simulink model "modeling1"  (R2017b)
settings: Solver=FixedStepAuto  StartTime=0.0  StopTime=100.0  FixedStep=0.01  RelTol=1e-3
settings Model: Creator=aokly  LastModifiedBy=aokly

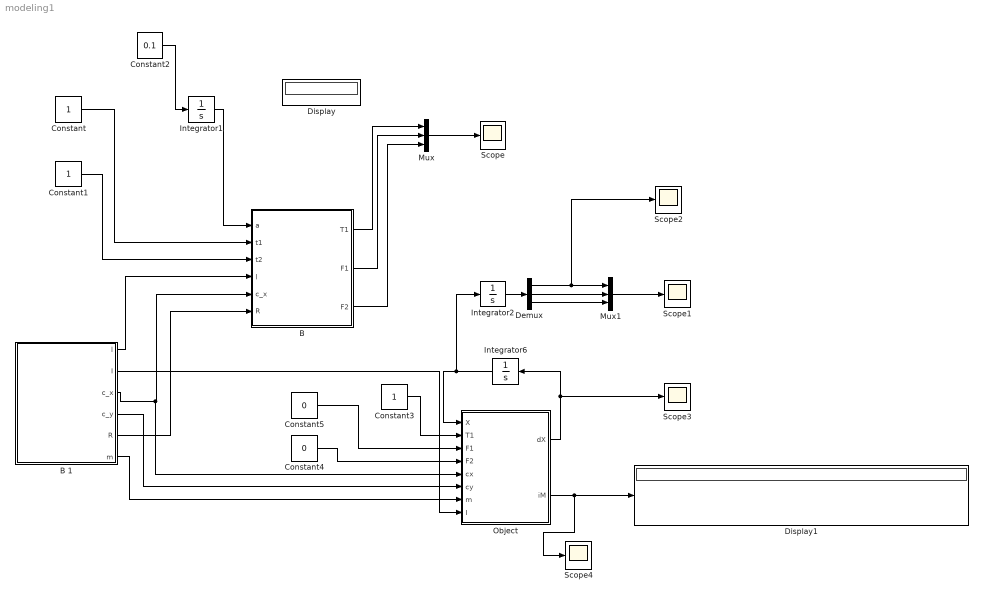
== system modeling1 ==
  "B " : MATLAB Function  TreatAsAtomicUnit=on
  B 1 : MATLAB Function  TreatAsAtomicUnit=on
  Constant : Constant
  Constant1 : Constant
  Constant2 : Constant  Value=0.1
  Constant3 : Constant
  Constant4 : Constant  Value=0
  Constant5 : Constant  Value=0
  Demux : Demux  Outputs=3
  Display : Display
  Display1 : Display
  Integrator1 : Integrator  InitialCondition=zeros(6,1)
  Integrator2 : Integrator  InitialCondition=zeros(3,1)
  Integrator6 : Integrator  InitialCondition=zeros(3,1)
  Mux : Mux  Inputs=3
  Mux1 : Mux  Inputs=3
  "Object " : MATLAB Function  TreatAsAtomicUnit=on
  Scope{,1..4} (5 alike) : Scope
  wires:
  Constant/1 -> "B "/2(t1)
  Constant1/1 -> "B "/3(t2)
  "B "/1(T1) -> Mux/1
  Mux/1 -> Scope/1
  B 1/1(l) -> "B "/4(l)
  B 1/3(c_x) -> "B "/5(c_x), "Object "/5(cx)
  B 1/5(R) -> "B "/6(R)
  "B "/3(F2) -> Mux/3
  "B "/2(F1) -> Mux/2
  Integrator6/1 -> Integrator2/1, "Object "/1(X)
  B 1/4(c_y) -> "Object "/6(cy)
  B 1/6(m) -> "Object "/7(m)
  B 1/2(I) -> "Object "/8(I)
  Demux/1 -> Scope2/1, Mux1/1
  Demux/2 -> Mux1/2
  Demux/3 -> Mux1/3
  Mux1/1 -> Scope1/1
  Constant2/1 -> Integrator1/1
  Integrator1/1 -> "B "/1(a)
  Constant3/1 -> "Object "/2(T1)
  Constant4/1 -> "Object "/4(F2)
  Constant5/1 -> "Object "/3(F1)
  "Object "/1(dX) -> Scope3/1, Integrator6/1
  "Object "/2(iM) -> Scope4/1, Display1/1
  Integrator2/1 -> Demux/1

== matlab function modeling1/B  ==
  data: a input; t1 input; T1 output; t2 input; F1 output; F2 output; l input; c_x input; R input
function [T1,F1,F2] = B(a,t1,t2,l,c_x,R)

V = [(l+c_x)*R	(l-c_x)*R;
	R*cos(a)    R*cos(a);
	R*sin(a) 	R*sin(a)]   *[t1;t2];


T1 = V(1);
F1 = V(2);
F2 = V(3);

end

== matlab function modeling1/Object  ==
  data: X input; T1 input; dX output; F1 input; F2 input; cx input; cy input; m input; I input; iM output
function [dX,iM] = fcn(X,T1,F1,F2,cx,cy,m,I)

dat = X(1);

A = [
[                             0,    (cx*dat)/(I + cy^2*m - cy^2),    (cy*dat)/(I + cy^2*m - cy^2)];
[ (cx*dat*(- cy^2 + I))/(cy^2*m^2 - cy^2*m + I*m) + (cx*cy^2*dat)/(I + cy^2*m - cy^2), (cx*cy*dat)/(I + cy^2*m - cy^2),  (cy^2*dat)/(I + cy^2*m - cy^2)];
[ (cy*dat*(I + cx^2*m + cy^2*m - cy^2))/(cy^2*m^2 - cy^2*m + I*m) - (cx^2*cy*dat)/(I + cy^2*m - cy^2),  (cx^2*dat)/(I + cy^2*m - cy^2), (cx*cy*dat)/(I + cy^2*m - cy^2)];
];


iM = [
[  -1/(I + cy^2*m - cy^2),                  cy/(I + cy^2*m - cy^2),                                 -cx/(I + cy^2*m - cy^2)];
[ -cy/(I + cy^2*m - cy^2), -(- cy^2 + I)/(cy^2*m^2 - cy^2*m + I*m),                            -(cx*cy)/(I + cy^2*m - cy^2)];
[ -cx/(I + cy^2*m - cy^2),             (cx*cy)/(I + cy^2*m - cy^2), -(I + cx^2*m + cy^2*m - cy^2)/(cy^2*m^2 - cy^2*m + I*m)];
];

%A = [zeros(6,3) [eye(3);zeros(3)]];
A = -eye(3);
dX = A*X+iM*[T1;F1;F2];
%disp(X);

%A*X+B*[T1;F1;F2]

== matlab function modeling1/B 1 ==
  data: l output; I output; c_x output; c_y output; R output; m output
function [l,I,c_x,c_y,R,m] = getConf()

l = 0.5;
I = 0.1;
c_x = 1;
c_y = 2;
R = 3;
m = 0.1;

end
